simulink model "hmapsf"  (R2020a)
settings: Solver=FixedStepAuto  StartTime=0.0  StopTime=1000000000000000000  FixedStep=tstep  RelTol=1e-3
model workspace (MAT data in the model file):
  IC_x0 = Simulink.Signal
  IC_x0.DataType = 'auto'
  IC_x0.Dimensions = -1
  IC_x0.DimensionsMode = 'auto'
  IC_x0.Complexity = 'auto'
  IC_x0.SampleTime = -1
  IC_x0.SamplingMode = 'auto'
  IC_x1 = Simulink.Signal
  IC_x1.DataType = 'auto'
  IC_x1.Dimensions = -1
  IC_x1.DimensionsMode = 'auto'
  IC_x1.Complexity = 'auto'
  IC_x1.SampleTime = -1
  IC_x1.SamplingMode = 'auto'
  IC_y1 = Simulink.Signal
  IC_y1.DataType = 'auto'
  IC_y1.Dimensions = -1
  IC_y1.DimensionsMode = 'auto'
  IC_y1.Complexity = 'auto'
  IC_y1.SampleTime = -1
  IC_y1.SamplingMode = 'auto'
  contsim_time = Simulink.Signal
  contsim_time.DataType = 'double'
  contsim_time.Dimensions = [1 1]
  contsim_time.DimensionsMode = 'auto'
  contsim_time.Complexity = 'real'
  contsim_time.SampleTime = -1
  contsim_time.SamplingMode = 'auto'
  ip = Simulink.Signal
  ip.DataType = 'double'
  ip.Dimensions = [1 2]
  ip.DimensionsMode = 'auto'
  ip.Complexity = 'auto'
  ip.SampleTime = -1
  ip.SamplingMode = 'auto'
  ip.InitialValue = '[0 0]'
  newnode = Simulink.Signal
  newnode.DataType = 'double'
  newnode.Dimensions = [1 2]
  newnode.DimensionsMode = 'auto'
  newnode.Complexity = 'real'
  newnode.SampleTime = -1
  newnode.SamplingMode = 'auto'
  newnode.InitialValue = '[0 0]'
  szxx1 = Simulink.Signal
  szxx1.DataType = 'double'
  szxx1.Dimensions = [1 1]
  szxx1.DimensionsMode = 'auto'
  szxx1.Complexity = 'real'
  szxx1.SampleTime = -1
  szxx1.SamplingMode = 'auto'
  szxx1.InitialValue = '0'
values from neighbouring files (symbols this model uses):
  H = struct    [hmapsf_Initializ.m]
  IC_theta0 = gamma_1+IC_theta1    (= 4.71238898038)    [hmapsf_Initializ.m]
  IC_theta1 = (3*pi)/2    (= 4.71238898038)    [hmapsf_Initializ.m]
  IC_x0 = IC_x0f-L_0f*cos(IC_theta0)    [hmapsf_Initializ.m]
  IC_x1 = 0    [hmapsf_Initializ.m]
  IC_y0 = IC_y0f-L_0f*sin(IC_theta0)    [hmapsf_Initializ.m]
  IC_y1 = 0    [hmapsf_Initializ.m]
  indsimtime = 300    [hmapsf_Initializ.m]
  L_0b = 0.48    [hmapsf_Initializ.m]
  L_0f = 3.8    [hmapsf_Initializ.m]
  L_1f = 7.21    [hmapsf_Initializ.m]
  LD = 10    [hmapsf_Initializ.m]
  tn = zeros(1,12)    [hmapsf_Initializ.m]
  tstep = 0.2    [hmapsf_Initializ.m]
undefined symbols (not defined in the file or in its folder): DiscIntNeverNeededParam
libraries: simulink x1
settings Model: PauseTimes=0  OrderedModelArguments=off  Creator=giridhar  LastModifiedBy=giridhar
settings SolverCC: AlgebraicLoopSolver=LineSearch
settings DebuggingCC: SFUnusedDataAndEventsDiag=none  UnderSpecifiedDimensionMsg=warning

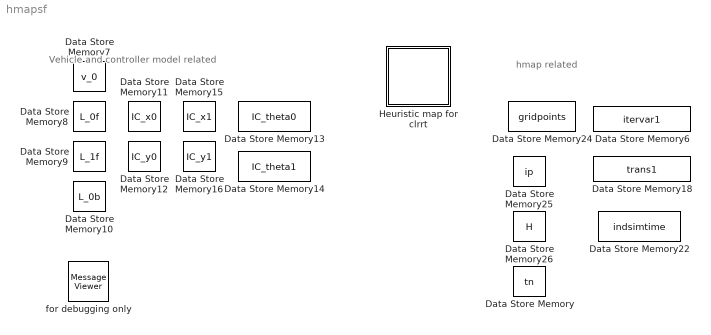
== system hmapsf ==
  note: Vehicle and controller model related
  note: hmap related
  Data Store Memory : DataStoreMemory  DataStoreName=tn  ReadBeforeWriteMsg=warning  WriteAfterWriteMsg=warning  WriteAfterReadMsg=warning  InitialValue=tn  VectorParams1D=off  ShowAdditionalParam=off  OutDataTypeStr=double
  Data Store Memory10 : DataStoreMemory  DataStoreName=L_0b  ReadBeforeWriteMsg=warning  WriteAfterWriteMsg=warning  WriteAfterReadMsg=warning  InitialValue=0.48  VectorParams1D=off  ShowAdditionalParam=off  OutDataTypeStr=double  Dimensions=[1 1]
  Data Store Memory11 : DataStoreMemory  DataStoreName=IC_x0  ReadBeforeWriteMsg=warning  WriteAfterWriteMsg=warning  WriteAfterReadMsg=warning  VectorParams1D=off  ShowAdditionalParam=off  OutDataTypeStr=double  Dimensions=[1 1]  StateMustResolveToSignalObject=on
  Data Store Memory12 : DataStoreMemory  DataStoreName=IC_y0  ReadBeforeWriteMsg=warning  WriteAfterWriteMsg=warning  WriteAfterReadMsg=warning  VectorParams1D=off  ShowAdditionalParam=off  OutDataTypeStr=double  Dimensions=[1 1]
  Data Store Memory13 : DataStoreMemory  DataStoreName=IC_theta0  ReadBeforeWriteMsg=warning  WriteAfterWriteMsg=warning  WriteAfterReadMsg=warning  VectorParams1D=off  ShowAdditionalParam=off  OutDataTypeStr=double  Dimensions=[1 1]
  Data Store Memory14 : DataStoreMemory  DataStoreName=IC_theta1  ReadBeforeWriteMsg=warning  WriteAfterWriteMsg=warning  WriteAfterReadMsg=warning  VectorParams1D=off  ShowAdditionalParam=off  OutDataTypeStr=double  Dimensions=[1 1]
  Data Store Memory15 : DataStoreMemory  DataStoreName=IC_x1  ReadBeforeWriteMsg=warning  WriteAfterWriteMsg=warning  WriteAfterReadMsg=warning  VectorParams1D=off  ShowAdditionalParam=off  OutDataTypeStr=double  Dimensions=[1 1]  StateMustResolveToSignalObject=on
  Data Store Memory16 : DataStoreMemory  DataStoreName=IC_y1  ReadBeforeWriteMsg=warning  WriteAfterWriteMsg=warning  WriteAfterReadMsg=warning  VectorParams1D=off  ShowAdditionalParam=off  OutDataTypeStr=double  Dimensions=[1 1]  StateMustResolveToSignalObject=on
  Data Store Memory18 : DataStoreMemory  DataStoreName=trans1  ReadBeforeWriteMsg=warning  WriteAfterWriteMsg=warning  WriteAfterReadMsg=warning  VectorParams1D=off  ShowAdditionalParam=off  OutDataTypeStr=double
  Data Store Memory22 : DataStoreMemory  DataStoreName=indsimtime  ReadBeforeWriteMsg=warning  WriteAfterWriteMsg=warning  WriteAfterReadMsg=warning  InitialValue=indsimtime  ShowAdditionalParam=off  OutDataTypeStr=double
  Data Store Memory24 : DataStoreMemory  DataStoreName=gridpoints  ReadBeforeWriteMsg=warning  WriteAfterWriteMsg=warning  WriteAfterReadMsg=warning  InitialValue=gridpoints  VectorParams1D=off  ShowAdditionalParam=off  OutDataTypeStr=double
  Data Store Memory25 : DataStoreMemory  DataStoreName=ip  ReadBeforeWriteMsg=warning  WriteAfterWriteMsg=warning  WriteAfterReadMsg=warning  InitialValue=[0 0]  VectorParams1D=off  ShowAdditionalParam=off  OutDataTypeStr=double  Dimensions=[1 2]  StateMustResolveToSignalObject=on
  Data Store Memory26 : DataStoreMemory  DataStoreName=H  ReadBeforeWriteMsg=warning  WriteAfterWriteMsg=warning  WriteAfterReadMsg=warning  InitialValue=H  VectorParams1D=off  ShowAdditionalParam=off  OutDataTypeStr=Bus: slBus1
  Data Store Memory6 : DataStoreMemory  DataStoreName=itervar1  ReadBeforeWriteMsg=warning  WriteAfterWriteMsg=warning  WriteAfterReadMsg=warning  VectorParams1D=off  ShowAdditionalParam=off  OutDataTypeStr=double
  Data Store Memory7 : DataStoreMemory  DataStoreName=v_0  ReadBeforeWriteMsg=warning  WriteAfterWriteMsg=warning  WriteAfterReadMsg=warning  InitialValue=v_0  VectorParams1D=off  ShowAdditionalParam=off  OutDataTypeStr=double  Dimensions=[1 1]
  Data Store Memory8 : DataStoreMemory  DataStoreName=L_0f  ReadBeforeWriteMsg=warning  WriteAfterWriteMsg=warning  WriteAfterReadMsg=warning  InitialValue=3.8  VectorParams1D=off  ShowAdditionalParam=off  OutDataTypeStr=double  Dimensions=[1 1]
  Data Store Memory9 : DataStoreMemory  DataStoreName=L_1f  ReadBeforeWriteMsg=warning  WriteAfterWriteMsg=warning  WriteAfterReadMsg=warning  InitialValue=7.21  VectorParams1D=off  ShowAdditionalParam=off  OutDataTypeStr=double  Dimensions=[1 1]
  Heuristic map for clrrt : Stateflow chart  TreatAsAtomicUnit=on
  for debugging only : MessageViewer  History=1000  SavedRootId=#

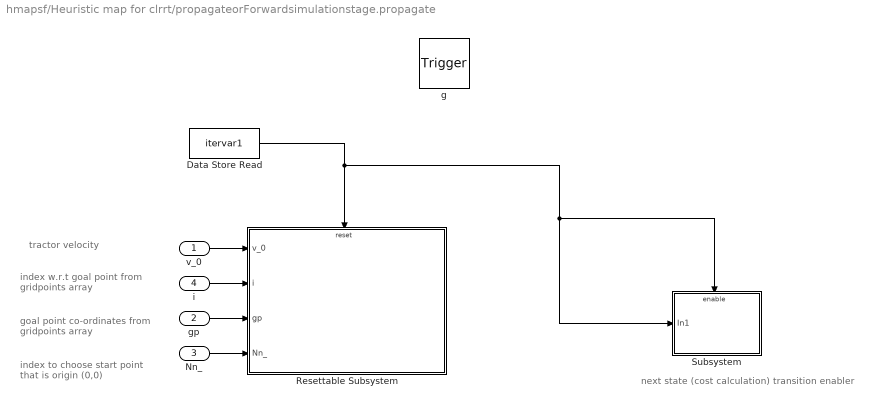
== system hmapsf/Heuristic map for clrrt/propagateorForwardsimulationstage.propagate ==
  note: index w.r.t goal point from
      | gridpoints array
  note: index to choose start point
      | that is origin (0,0)
  note: goal point co-ordinates from
      | gridpoints array
  note: tractor velocity
  note: next state (cost calculation) transition enabler
  v_0 : Inport  OutDataTypeStr=double  PortDimensions=1
  gp : Inport  Port=2  OutMin=1  OutMax=2  OutDataTypeStr=double  PortDimensions=[1 3]
  Nn_ : Inport  Port=3  OutDataTypeStr=double  PortDimensions=1
  i : Inport  Port=4  OutDataTypeStr=double  PortDimensions=1
  g : TriggerPort  TriggerType=function-call  VariantControl=(inherit)  SampleTime=0.2
      settings: CopyFcn=Stateflow.SLINSF.SimulinkMan.removeBlockPreDeleteFcn  PreDeleteFcn=Stateflow.SLINSF.SimulinkMan.unsafePredeleteFcn
  Data Store Read : DataStoreRead  DataStoreName=itervar1
  Resettable Subsystem : Subsystem  Priority=1  TreatAsAtomicUnit=on
  Subsystem : Subsystem  Priority=2
  wires:
  gp/1 -> Resettable Subsystem/3(gp)
  v_0/1 -> Resettable Subsystem/1(v_0)
  Nn_/1 -> Resettable Subsystem/4(Nn_)
  i/1 -> Resettable Subsystem/2(i)
  Data Store Read/1 -> Subsystem/Enable, Subsystem/1(In1), Resettable Subsystem/Reset

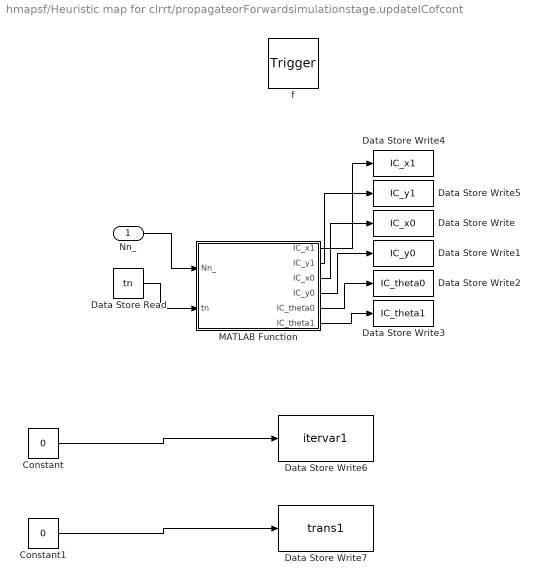
== system hmapsf/Heuristic map for clrrt/propagateorForwardsimulationstage.updateICofcont ==
  Nn_ : Inport  OutDataTypeStr=double  PortDimensions=1
  f : TriggerPort  TriggerType=function-call  VariantControl=(inherit)
      settings: CopyFcn=Stateflow.SLINSF.SimulinkMan.removeBlockPreDeleteFcn  PreDeleteFcn=Stateflow.SLINSF.SimulinkMan.unsafePredeleteFcn
  Constant : Constant  Value=0
  Constant1 : Constant  Value=0
  Data Store Read : DataStoreRead  DataStoreName=tn
  Data Store Write : DataStoreWrite  DataStoreName=IC_x0
  Data Store Write1 : DataStoreWrite  DataStoreName=IC_y0
  Data Store Write2 : DataStoreWrite  DataStoreName=IC_theta0
  Data Store Write3 : DataStoreWrite  DataStoreName=IC_theta1
  Data Store Write4 : DataStoreWrite  DataStoreName=IC_x1
  Data Store Write5 : DataStoreWrite  DataStoreName=IC_y1
  Data Store Write6 : DataStoreWrite  DataStoreName=itervar1
  Data Store Write7 : DataStoreWrite  DataStoreName=trans1
  MATLAB Function : MATLAB Function  TreatAsAtomicUnit=on
  wires:
  Nn_/1 -> MATLAB Function/1(Nn_)
  Data Store Read/1 -> MATLAB Function/2(tn)
  MATLAB Function/6(IC_theta1) -> Data Store Write3/1
  MATLAB Function/5(IC_theta0) -> Data Store Write2/1
  MATLAB Function/4(IC_y0) -> Data Store Write1/1
  MATLAB Function/3(IC_x0) -> Data Store Write/1
  MATLAB Function/2(IC_y1) -> Data Store Write5/1
  MATLAB Function/1(IC_x1) -> Data Store Write4/1
  Constant/1 -> Data Store Write6/1
  Constant1/1 -> Data Store Write7/1

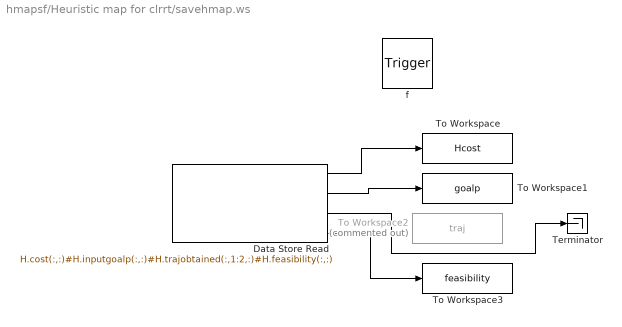
== system hmapsf/Heuristic map for clrrt/savehmap.ws ==
  f : TriggerPort  TriggerType=function-call  VariantControl=(inherit)
      settings: CopyFcn=Stateflow.SLINSF.SimulinkMan.removeBlockPreDeleteFcn  PreDeleteFcn=Stateflow.SLINSF.SimulinkMan.unsafePredeleteFcn
  Data Store Read : DataStoreRead  DataStoreName=H  DataStoreElements=H.cost(:,:)#H.inputgoalp(:,:)#H.trajobtained(:,1:2,:)#H.feasibility(:,:)
  Terminator : Terminator
  To Workspace : ToWorkspace  VariableName=Hcost  SaveFormat=Structure  SampleTime=-1
  To Workspace1 : ToWorkspace  VariableName=goalp  SaveFormat=Timeseries  SampleTime=-1
  To Workspace2 : ToWorkspace  Commented=on  VariableName=traj  SaveFormat=Structure  SampleTime=-1
  To Workspace3 : ToWorkspace  VariableName=feasibility  SaveFormat=Structure  SampleTime=-1
  wires:
  Data Store Read/1 -> To Workspace/1
  Data Store Read/2 -> To Workspace1/1
  Data Store Read/3 -> Terminator/1
  Data Store Read/4 -> To Workspace3/1

== system hmapsf/Heuristic map for clrrt/stop ==
  f : TriggerPort  TriggerType=function-call  VariantControl=(inherit)
      settings: CopyFcn=Stateflow.SLINSF.SimulinkMan.removeBlockPreDeleteFcn  PreDeleteFcn=Stateflow.SLINSF.SimulinkMan.unsafePredeleteFcn
  Constant : Constant
  Stop Simulation : Stop
  wires:
  Constant/1 -> Stop Simulation/1

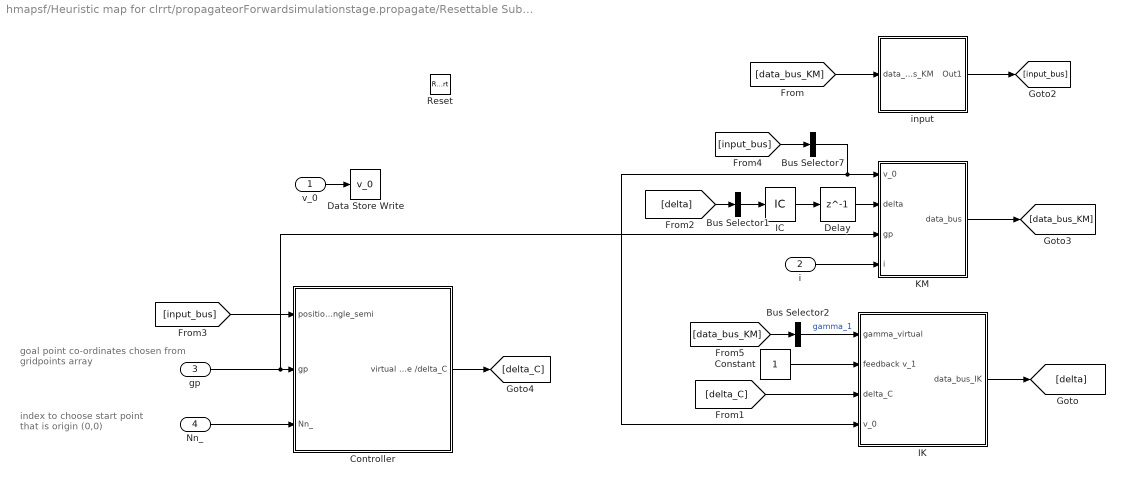
== system hmapsf/Heuristic map for clrrt/propagateorForwardsimulationstage.propagate/Resettable Subsystem ==
  note: goal point co-ordinates chosen from
      | gridpoints array
  note: index to choose start point
      | that is origin (0,0)
  v_0 : Inport  OutDataTypeStr=double  PortDimensions=1
  i : Inport  Port=2  OutDataTypeStr=double  PortDimensions=1
  gp : Inport  Port=3  OutMin=1  OutMax=2  OutDataTypeStr=double  PortDimensions=[1 3]
  Nn_ : Inport  Port=4  OutDataTypeStr=double  PortDimensions=1
  Reset : ResetPort  DisableCoverage=on  ResetTriggerType=level  PropagateVarSize=During execution
  Bus Selector1 : BusSelector  OutputSignals=angle.steering_angle  OutputAsBus=on
  Bus Selector2 : BusSelector  OutputSignals=angle.articulation_angle  OutputAsBus=on
  Bus Selector7 : BusSelector  OutputSignals=u_0  OutputAsBus=on
  Constant : Constant
  Controller : Subsystem
  Data Store Write : DataStoreWrite  DataStoreName=v_0
  Delay : Delay  DelayLength=1
  IC : InitialCondition  Value=0
  IK : Subsystem  SystemSampleTime=0.8
  KM : Subsystem  SystemSampleTime=0.8
  input : Subsystem
  wires:
  [data_bus_KM] -> Bus Selector2/1
  input/1(Out1) -> [input_bus]
  [delta_C] -> IK/3(delta_C)
  Bus Selector7/1 -> IK/4(v_0), KM/1(v_0)
  [delta] -> Bus Selector1/1
  Nn_/1 -> Controller/3(Nn_)
  i/1 -> KM/4(i)
  Delay/1 -> KM/2(delta)
  Constant/1 -> IK/2(feedback v_1)
  IC/1 -> Delay/1
  KM/1(data_bus) -> [data_bus_KM]
  Bus Selector2/1 -> IK/1(gamma_virtual)  "gamma_1"
  Bus Selector1/1 -> IC/1
  v_0/1 -> Data Store Write/1
  IK/1(data_bus_IK) -> [delta]
  [input_bus] -> Bus Selector7/1
  [data_bus_KM] -> input/1(data_bus_KM)
  [input_bus] -> Controller/1(positions_yawangle_semi)
  gp/1 -> Controller/2(gp), KM/3(gp)
  Controller/1(virtual steer angle /delta_C) -> [delta_C]

== system hmapsf/Heuristic map for clrrt/propagateorForwardsimulationstage.propagate/Subsystem ==
  In1 : Inport
  Enable : EnablePort  StatesWhenEnabling=reset
  Subsystem : Subsystem  Priority=2
  wires:
  In1/1 -> Subsystem/1(In1)

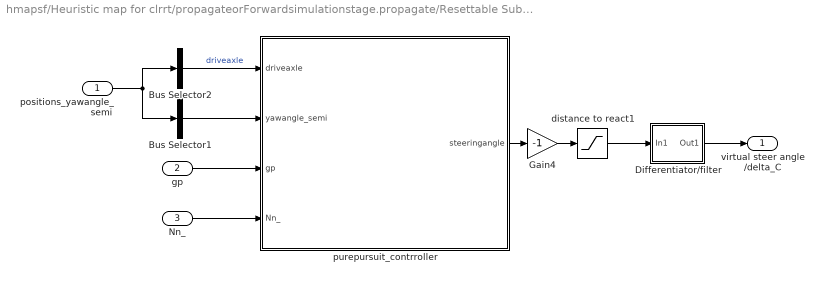
== system hmapsf/Heuristic map for clrrt/propagateorForwardsimulationstage.propagate/Resettable Subsystem/Controller ==
  positions_yawangle_semi : Inport
  gp : Inport  Port=2
  Nn_ : Inport  Port=3
  Bus Selector1 : BusSelector  OutputSignals=yawangle_semi  OutputAsBus=on
  Bus Selector2 : BusSelector  OutputSignals=positions  OutputAsBus=on
  Differentiator/filter : Subsystem  mask{ts=13.5}
      mask prompts: ts "response_time"
      mask init:
      | c=(3*pi/ts)^2;
  Gain4 : Gain  Gain=-1
  distance to react1 : Saturate  UpperLimit=1  LowerLimit=-1
  purepursuit_contrroller : Subsystem
  virtual steer angle /delta_C : Outport  PortDimensions=[1,1]  VectorParamsAs1DForOutWhenUnconnected=off
  wires:
  distance to react1/1 -> Differentiator/filter/1(In1)
  purepursuit_contrroller/1(steeringangle) -> Gain4/1
  Bus Selector2/1 -> purepursuit_contrroller/1(driveaxle)  "driveaxle"
  positions_yawangle_semi/1 -> Bus Selector1/1, Bus Selector2/1
  gp/1 -> purepursuit_contrroller/3(gp)
  Nn_/1 -> purepursuit_contrroller/4(Nn_)
  Gain4/1 -> distance to react1/1
  Bus Selector1/1 -> purepursuit_contrroller/2(yawangle_semi)
  Differentiator/filter/1(Out1) -> virtual steer angle /delta_C/1

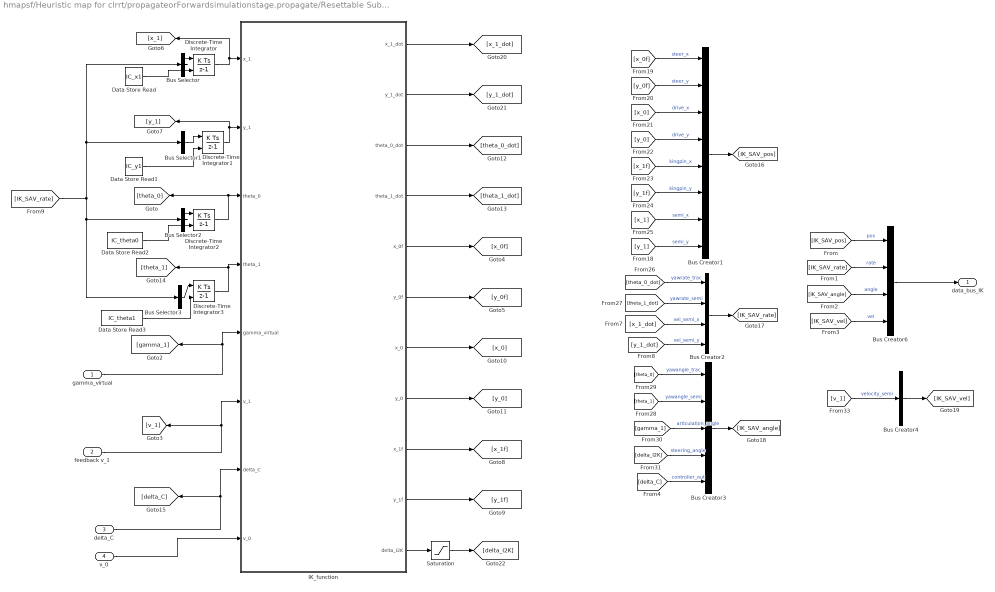
== system hmapsf/Heuristic map for clrrt/propagateorForwardsimulationstage.propagate/Resettable Subsystem/IK ==
  gamma_virtual : Inport
  feedback v_1 : Inport  Port=2
  delta_C : Inport  Port=3
  v_0 : Inport  Port=4
  Bus Creator1 : BusCreator  Inputs=8
  Bus Creator2 : BusCreator  Inputs=4
  Bus Creator3 : BusCreator  Inputs=5
  Bus Creator4 : BusCreator  Inputs=1
  Bus Creator6 : BusCreator  Inputs=4
  Bus Selector : BusSelector  OutputSignals=vel_semi_x  OutputAsBus=on
  Bus Selector1 : BusSelector  OutputSignals=vel_semi_y  OutputAsBus=on
  Bus Selector2 : BusSelector  OutputSignals=yawrate_trac  OutputAsBus=on
  Bus Selector3 : BusSelector  OutputSignals=yawrate_semi  OutputAsBus=on
  Data Store Read : DataStoreRead  DataStoreName=IC_x1
  Data Store Read1 : DataStoreRead  DataStoreName=IC_y1
  Data Store Read2 : DataStoreRead  DataStoreName=IC_theta0
  Data Store Read3 : DataStoreRead  DataStoreName=IC_theta1
  Discrete-Time Integrator : DiscreteIntegrator  InitialConditionSource=external  InitialCondition=IC_x1  SampleTime=-1  ICPrevOutput=DiscIntNeverNeededParam  ICPrevScaledInput=DiscIntNeverNeededParam
  Discrete-Time Integrator1 : DiscreteIntegrator  InitialConditionSource=external  InitialCondition=IC_y1  SampleTime=-1  ICPrevOutput=DiscIntNeverNeededParam  ICPrevScaledInput=DiscIntNeverNeededParam
  Discrete-Time Integrator2 : DiscreteIntegrator  InitialConditionSource=external  InitialCondition=IC_theta0  SampleTime=-1  ICPrevOutput=DiscIntNeverNeededParam  ICPrevScaledInput=DiscIntNeverNeededParam
  Discrete-Time Integrator3 : DiscreteIntegrator  InitialConditionSource=external  InitialCondition=IC_theta1  SampleTime=-1  ICPrevOutput=DiscIntNeverNeededParam  ICPrevScaledInput=DiscIntNeverNeededParam
  IK_function : MATLAB Function  TreatAsAtomicUnit=on
  Saturation : Saturate  UpperLimit=0.7  LowerLimit=-0.7
  data_bus_IK : Outport  VectorParamsAs1DForOutWhenUnconnected=off
  wires:
  IK_function/7(x_0) -> [x_0]
  IK_function/8(y_0) -> [y_0]
  IK_function/1(x_1_dot) -> [x_1_dot]
  IK_function/3(theta_0_dot) -> [theta_0_dot]
  IK_function/4(theta_1_dot) -> [theta_1_dot]
  IK_function/10(y_1f) -> [y_1f]
  IK_function/9(x_1f) -> [x_1f]
  Discrete-Time Integrator/1 -> [x_1], IK_function/1(x_1)
  Discrete-Time Integrator1/1 -> [y_1], IK_function/2(y_1)
  gamma_virtual/1 -> [gamma_1], IK_function/5(gamma_virtual)
  IK_function/2(y_1_dot) -> [y_1_dot]
  Discrete-Time Integrator3/1 -> IK_function/4(theta_1), [theta_1]
  IK_function/5(x_0f) -> [x_0f]
  IK_function/6(y_0f) -> [y_0f]
  [y_0f] -> Bus Creator1/2  "steer_y"
  [x_1f] -> Bus Creator1/5  "kingpin_x"
  Bus Creator6/1 -> data_bus_IK/1
  [v_1] -> Bus Creator4/1  "velocity_semi"
  [x_0] -> Bus Creator1/3  "drive_x"
  [y_1f] -> Bus Creator1/6  "kingpin_y"
  [x_0f] -> Bus Creator1/1  "steer_x"
  [y_0] -> Bus Creator1/4  "drive_y"
  Bus Creator3/1 -> [IK_SAV_angle]
  [theta_0_dot] -> Bus Creator2/1  "yawrate_trac"
  [theta_1_dot] -> Bus Creator2/2  "yawrate_semi"
  Discrete-Time Integrator2/1 -> [theta_0], IK_function/3(theta_0)
  [IK_SAV_rate] -> Bus Selector/1, Bus Selector1/1, Bus Selector3/1, Bus Selector2/1
  Bus Creator2/1 -> [IK_SAV_rate]
  Bus Creator1/1 -> [IK_SAV_pos]
  [delta_I2K] -> Bus Creator3/4  "steering_angle"
  [gamma_1] -> Bus Creator3/3  "articulation_angle"
  Bus Creator4/1 -> [IK_SAV_vel]
  [theta_1] -> Bus Creator3/2  "yawangle_semi"
  [IK_SAV_rate] -> Bus Creator6/2  "rate"
  [theta_0] -> Bus Creator3/1  "yawangle_trac"
  [IK_SAV_pos] -> Bus Creator6/1  "pos"
  [IK_SAV_angle] -> Bus Creator6/3  "angle"
  [IK_SAV_vel] -> Bus Creator6/4  "vel"
  Bus Selector3/1 -> Discrete-Time Integrator3/1
  Bus Selector2/1 -> Discrete-Time Integrator2/1
  Bus Selector/1 -> Discrete-Time Integrator/1
  Bus Selector1/1 -> Discrete-Time Integrator1/1
  [y_1_dot] -> Bus Creator2/4  "vel_semi_y"
  [x_1_dot] -> Bus Creator2/3  "vel_semi_x"
  IK_function/11(delta_I2K) -> Saturation/1
  [delta_C] -> Bus Creator3/5  "controller_out"
  feedback v_1/1 -> [v_1], IK_function/6(v_1)
  Saturation/1 -> [delta_I2K]
  [y_1] -> Bus Creator1/8  "semi_y"
  [x_1] -> Bus Creator1/7  "semi_x"
  Data Store Read3/1 -> Discrete-Time Integrator3/2
  Data Store Read2/1 -> Discrete-Time Integrator2/2
  Data Store Read1/1 -> Discrete-Time Integrator1/2
  Data Store Read/1 -> Discrete-Time Integrator/2
  v_0/1 -> IK_function/8(v_0)
  delta_C/1 -> IK_function/7(delta_C), [delta_C]

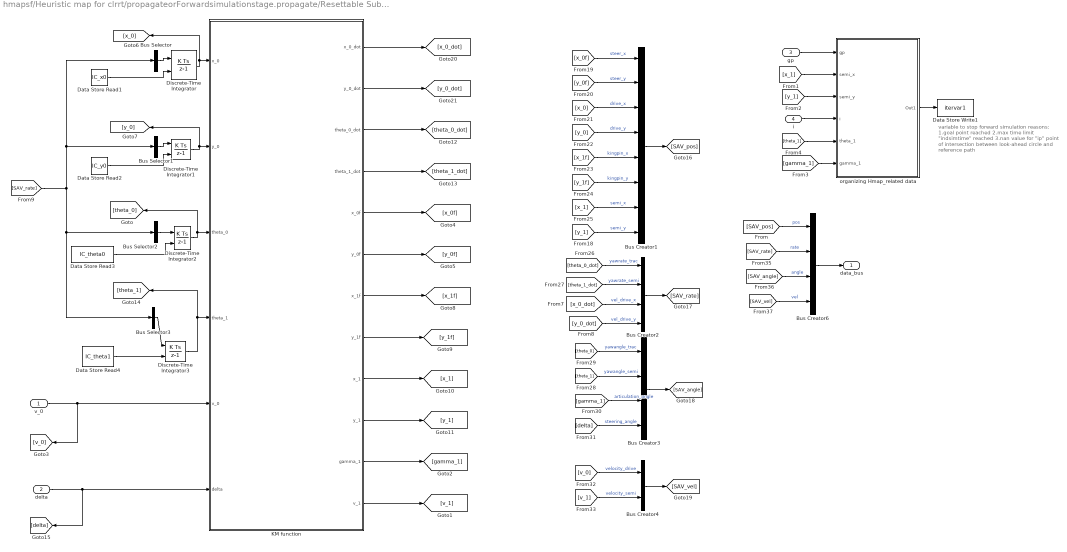
== system hmapsf/Heuristic map for clrrt/propagateorForwardsimulationstage.propagate/Resettable Subsystem/KM ==
  note: variable to stop forward simulation
      | reasons:
      | 1.goal point reached
      | 2.max time limit "indsimtime" reached
      | 3.nan value for "ip" point of intersection
      | between look-ahead circle and reference path
  v_0 : Inport
  delta : Inport  Port=2
  gp : Inport  Port=3
  i : Inport  Port=4  OutDataTypeStr=double
  Bus Creator1 : BusCreator  Inputs=8
  Bus Creator2 : BusCreator  Inputs=4
  Bus Creator3 : BusCreator  Inputs=4
  Bus Creator4 : BusCreator  Inputs=2
  Bus Creator6 : BusCreator  Inputs=4
  Bus Selector : BusSelector  OutputSignals=vel_drive_x  OutputAsBus=on
  Bus Selector1 : BusSelector  OutputSignals=vel_drive_y  OutputAsBus=on
  Bus Selector2 : BusSelector  OutputSignals=yawrate_trac  OutputAsBus=on
  Bus Selector3 : BusSelector  OutputSignals=yawrate_semi  OutputAsBus=on
  Data Store Read1 : DataStoreRead  DataStoreName=IC_x0
  Data Store Read2 : DataStoreRead  DataStoreName=IC_y0
  Data Store Read3 : DataStoreRead  DataStoreName=IC_theta0
  Data Store Read4 : DataStoreRead  DataStoreName=IC_theta1
  Data Store Write1 : DataStoreWrite  DataStoreName=itervar1
  Discrete-Time Integrator : DiscreteIntegrator  InitialConditionSource=external  InitialCondition=IC_x0  SampleTime=-1  ICPrevOutput=DiscIntNeverNeededParam  ICPrevScaledInput=DiscIntNeverNeededParam
  Discrete-Time Integrator1 : DiscreteIntegrator  InitialConditionSource=external  InitialCondition=IC_y0  SampleTime=-1  ICPrevOutput=DiscIntNeverNeededParam  ICPrevScaledInput=DiscIntNeverNeededParam
  Discrete-Time Integrator2 : DiscreteIntegrator  InitialConditionSource=external  InitialCondition=IC_theta0  SampleTime=-1  ICPrevOutput=DiscIntNeverNeededParam  ICPrevScaledInput=DiscIntNeverNeededParam
  Discrete-Time Integrator3 : DiscreteIntegrator  InitialConditionSource=external  InitialCondition=IC_theta1  SampleTime=-1  ICPrevOutput=DiscIntNeverNeededParam  ICPrevScaledInput=DiscIntNeverNeededParam
  KM function : MATLAB Function  TreatAsAtomicUnit=on
  "organizing Hmap_related data " : Subsystem
  data_bus : Outport  VectorParamsAs1DForOutWhenUnconnected=off
  wires:
  KM function/9(x_1) -> [x_1]
  KM function/10(y_1) -> [y_1]
  KM function/1(x_0_dot) -> [x_0_dot]
  KM function/3(theta_0_dot) -> [theta_0_dot]
  KM function/4(theta_1_dot) -> [theta_1_dot]
  KM function/8(y_1f) -> [y_1f]
  KM function/7(x_1f) -> [x_1f]
  Discrete-Time Integrator/1 -> KM function/1(x_0), [x_0]
  Discrete-Time Integrator1/1 -> KM function/2(y_0), [y_0]
  KM function/11(gamma_1) -> [gamma_1]
  KM function/2(y_0_dot) -> [y_0_dot]
  delta/1 -> [delta], KM function/6(delta)
  Discrete-Time Integrator3/1 -> [theta_1], KM function/4(theta_1)
  KM function/5(x_0f) -> [x_0f]
  KM function/6(y_0f) -> [y_0f]
  v_0/1 -> [v_0], KM function/5(v_0)
  [y_0f] -> Bus Creator1/2  "steer_y"
  [x_1f] -> Bus Creator1/5  "kingpin_x"
  Bus Creator6/1 -> data_bus/1
  [v_1] -> Bus Creator4/2  "velocity_semi"
  [x_0] -> Bus Creator1/3  "drive_x"
  [y_1f] -> Bus Creator1/6  "kingpin_y"
  [x_0f] -> Bus Creator1/1  "steer_x"
  [y_0] -> Bus Creator1/4  "drive_y"
  Bus Creator3/1 -> [SAV_angle]
  [v_0] -> Bus Creator4/1  "velocity_drive"
  [theta_0_dot] -> Bus Creator2/1  "yawrate_trac"
  [theta_1_dot] -> Bus Creator2/2  "yawrate_semi"
  Discrete-Time Integrator2/1 -> [theta_0], KM function/3(theta_0)
  [SAV_rate] -> Bus Selector/1, Bus Selector1/1, Bus Selector3/1, Bus Selector2/1
  Bus Creator2/1 -> [SAV_rate]
  Bus Creator1/1 -> [SAV_pos]
  [delta] -> Bus Creator3/4  "steering_angle"
  [gamma_1] -> Bus Creator3/3  "articulation_angle"
  Bus Creator4/1 -> [SAV_vel]
  [theta_1] -> Bus Creator3/2  "yawangle_semi"
  [SAV_rate] -> Bus Creator6/2  "rate"
  [theta_0] -> Bus Creator3/1  "yawangle_trac"
  [SAV_pos] -> Bus Creator6/1  "pos"
  [SAV_angle] -> Bus Creator6/3  "angle"
  [SAV_vel] -> Bus Creator6/4  "vel"
  Bus Selector3/1 -> Discrete-Time Integrator3/1
  Bus Selector2/1 -> Discrete-Time Integrator2/1
  Bus Selector/1 -> Discrete-Time Integrator/1
  Bus Selector1/1 -> Discrete-Time Integrator1/1
  [y_0_dot] -> Bus Creator2/4  "vel_drive_y"
  [x_0_dot] -> Bus Creator2/3  "vel_drive_x"
  KM function/12(v_1) -> [v_1]
  [x_1] -> Bus Creator1/7  "semi_x"
  [y_1] -> Bus Creator1/8  "semi_y"
  Data Store Read4/1 -> Discrete-Time Integrator3/2
  Data Store Read2/1 -> Discrete-Time Integrator1/2
  Data Store Read3/1 -> Discrete-Time Integrator2/2
  gp/1 -> "organizing Hmap_related data "/1(gp)
  i/1 -> "organizing Hmap_related data "/4(i)
  "organizing Hmap_related data "/1(Out1) -> Data Store Write1/1
  [theta_1] -> "organizing Hmap_related data "/5(theta_1)
  [y_1] -> "organizing Hmap_related data "/3(semi_y)
  [x_1] -> "organizing Hmap_related data "/2(semi_x)
  [gamma_1] -> "organizing Hmap_related data "/6(gamma_1)
  Data Store Read1/1 -> Discrete-Time Integrator/2

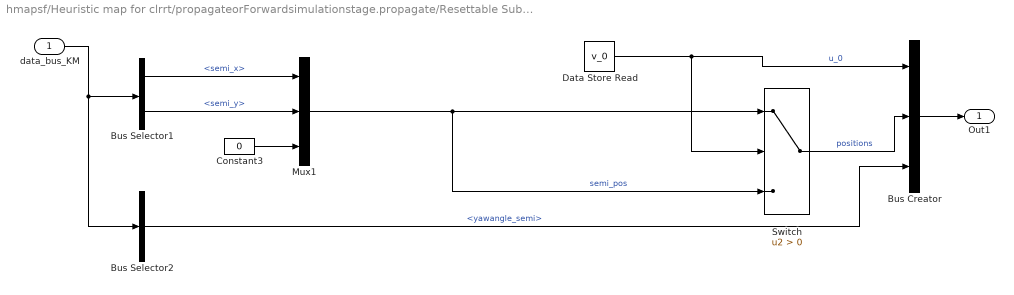
== system hmapsf/Heuristic map for clrrt/propagateorForwardsimulationstage.propagate/Resettable Subsystem/input ==
  data_bus_KM : Inport
  Bus Creator : BusCreator  Inputs=3
  Bus Selector1 : BusSelector  OutputSignals=pos.semi_x,pos.semi_y
  Bus Selector2 : BusSelector  OutputSignals=angle.yawangle_semi
  Constant3 : Constant  Value=0
  Data Store Read : DataStoreRead  DataStoreName=v_0
  Mux1 : Mux  Inputs=3
  Switch : Switch  Criteria=u2 > Threshold
  Out1 : Outport  VectorParamsAs1DForOutWhenUnconnected=off
  wires:
  Data Store Read/1 -> Switch/2, Bus Creator/1  "u_0"
  Bus Creator/1 -> Out1/1
  Constant3/1 -> Mux1/3
  data_bus_KM/1 -> Bus Selector2/1, Bus Selector1/1
  Bus Selector1/1 -> Mux1/1  "<semi_x>"
  Bus Selector1/2 -> Mux1/2  "<semi_y>"
  Mux1/1 -> Switch/1, Switch/3  "semi_pos"
  Switch/1 -> Bus Creator/2  "positions"
  Bus Selector2/1 -> Bus Creator/3  "<yawangle_semi>"

== system hmapsf/Heuristic map for clrrt/propagateorForwardsimulationstage.propagate/Subsystem/Subsystem ==
  note: variable for the stateflow transition condition
      | lets the control flow from forward simulation to cost calculation
      | in stateflow chart
  In1 : Inport
  Data Store Write : DataStoreWrite  DataStoreName=trans1
  wires:
  In1/1 -> Data Store Write/1

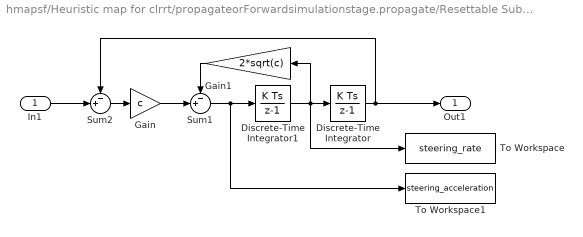
== system hmapsf/Heuristic map for clrrt/propagateorForwardsimulationstage.propagate/Resettable Subsystem/Controller/Differentiator//filter ==
  In1 : Inport
  Discrete-Time Integrator : DiscreteIntegrator  SampleTime=-1  ICPrevOutput=DiscIntNeverNeededParam  ICPrevScaledInput=DiscIntNeverNeededParam
  Discrete-Time Integrator1 : DiscreteIntegrator  SampleTime=-1  ICPrevOutput=DiscIntNeverNeededParam  ICPrevScaledInput=DiscIntNeverNeededParam
  Gain : Gain  Gain=c  SaturateOnIntegerOverflow=on  OutDataTypeStr=Inherit: Same as input  ParamDataTypeStr=Inherit: Same as input
  Gain1 : Gain  Gain=2*sqrt(c)  SaturateOnIntegerOverflow=on  OutDataTypeStr=Inherit: Same as input  ParamDataTypeStr=Inherit: Same as input
  Sum1 : Sum  Inputs=-+|  SaturateOnIntegerOverflow=on
  Sum2 : Sum  Inputs=-+|  SaturateOnIntegerOverflow=on
  To Workspace : ToWorkspace  VariableName=steering_rate  SampleTime=-1
  To Workspace1 : ToWorkspace  VariableName=steering_acceleration  SampleTime=-1
  Out1 : Outport
  wires:
  Discrete-Time Integrator1/1 -> Discrete-Time Integrator/1, To Workspace/1, Gain1/1
  Discrete-Time Integrator/1 -> Out1/1, Sum2/1
  Sum1/1 -> Discrete-Time Integrator1/1, To Workspace1/1
  Sum2/1 -> Gain/1
  In1/1 -> Sum2/2
  Gain1/1 -> Sum1/1
  Gain/1 -> Sum1/2

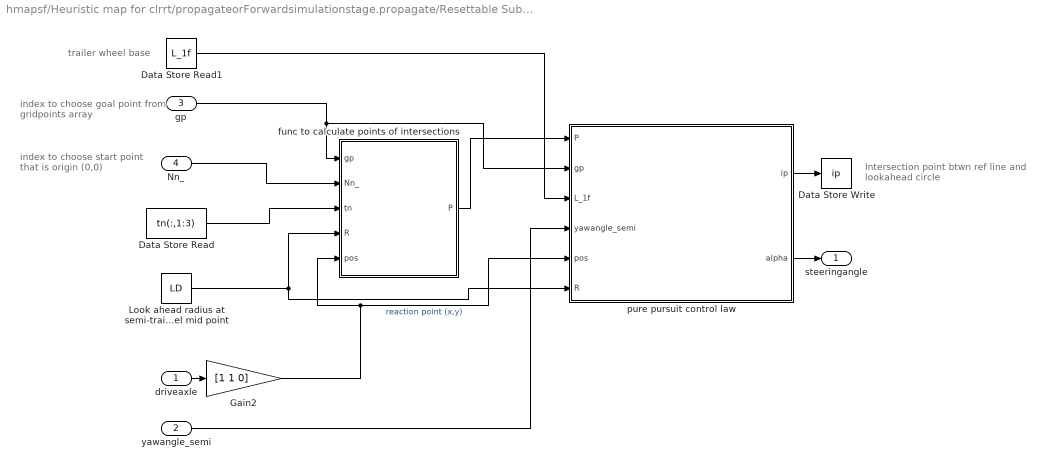
== system hmapsf/Heuristic map for clrrt/propagateorForwardsimulationstage.propagate/Resettable Subsystem/Controller/purepursuit_contrroller ==
  note: index to choose goal point from
      | gridpoints array
  note: trailer wheel base
  note: Intersection point
      | btwn ref line and lookahead circle
  note: index to choose start point
      | that is origin (0,0)
  driveaxle : Inport
  yawangle_semi : Inport  Port=2
  gp : Inport  Port=3
  Nn_ : Inport  Port=4
  Data Store Read : DataStoreRead  DataStoreName=tn  DataStoreElements=tn(:,1:3)
  Data Store Read1 : DataStoreRead  DataStoreName=L_1f
  Data Store Write : DataStoreWrite  DataStoreName=ip
  Gain2 : Gain  Gain=[1 1 0]
  Look ahead radius at semi-trailer axel mid point : Constant  Value=LD
  func to calculate points of intersections : MATLAB Function  TreatAsAtomicUnit=on
  pure pursuit control law : MATLAB Function  TreatAsAtomicUnit=on
  steeringangle : Outport  VectorParamsAs1DForOutWhenUnconnected=off
  wires:
  Data Store Read1/1 -> pure pursuit control law/3(L_1f)
  func to calculate points of intersections/1(P) -> pure pursuit control law/1(P)
  pure pursuit control law/1(ip) -> Data Store Write/1
  Look ahead radius at semi-trailer axel mid point/1 -> func to calculate points of intersections/4(R), pure pursuit control law/6(R)
  pure pursuit control law/2(alpha) -> steeringangle/1
  gp/1 -> func to calculate points of intersections/1(gp), pure pursuit control law/2(gp)
  Gain2/1 -> func to calculate points of intersections/5(pos), pure pursuit control law/5(pos)  "reaction point (x,y)"
  driveaxle/1 -> Gain2/1
  yawangle_semi/1 -> pure pursuit control law/4(yawangle_semi)
  Nn_/1 -> func to calculate points of intersections/2(Nn_)
  Data Store Read/1 -> func to calculate points of intersections/3(tn)

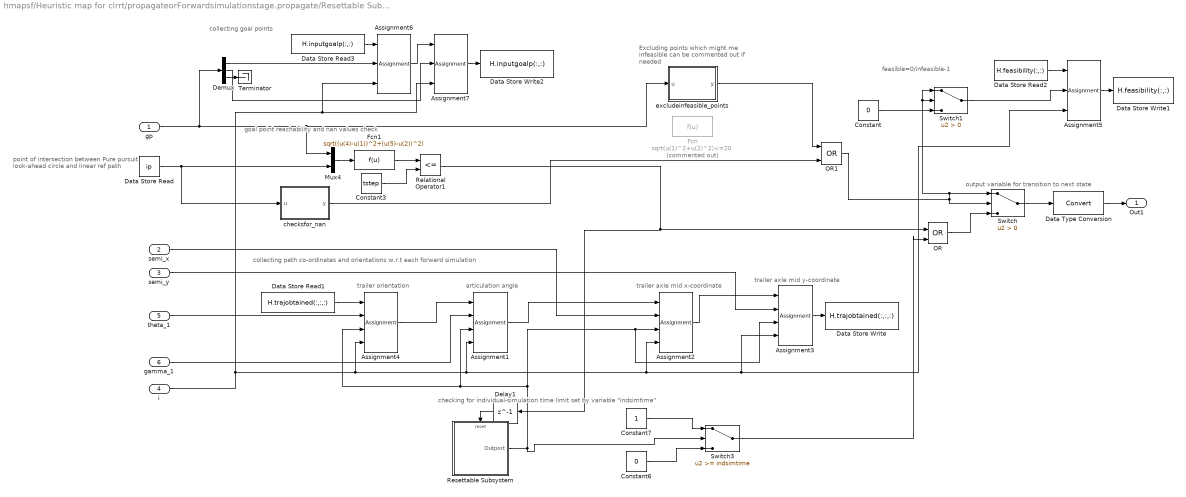
== system hmapsf/Heuristic map for clrrt/propagateorForwardsimulationstage.propagate/Resettable Subsystem/KM/organizing Hmap_related data  ==
  note: checking for individual simulation time limit set by variable "indsimtime"
  note: output variable for transition to next state
  note: Excluding points which might me infeasible can be commented out if needed
  note: collecting path co-ordinates and orientations w.r.t each forward simulation
  note: goal point reachability and nan values check
  note: point of intersection between Pure pursuit
      | look-ahead circle and linear ref path
  note: collecting goal points
  note: feasible=0/infeasible-1
  note: trailer axle mid x-coordinate
  note: trailer orientation
  note: articulation angle
  note: trailer axle mid y-coordinate
  gp : Inport  PortDimensions=[1 3]
  semi_x : Inport  Port=2
  semi_y : Inport  Port=3
  i : Inport  Port=4  OutDataTypeStr=double
  theta_1 : Inport  Port=5
  gamma_1 : Inport  Port=6  OutDataTypeStr=double  PortDimensions=1
  Assignment1 : Assignment  NumberOfDimensions=3  DiagnosticForDimensions=Warning  IndexOptions=Index vector (port),Index vector (dialog),Index vector (port)  Indices=1,4,1  OutputSizes=1,1,1
  Assignment2 : Assignment  NumberOfDimensions=3  DiagnosticForDimensions=Warning  IndexOptions=Index vector (port),Index vector (dialog),Index vector (port)  Indices=1,1,1  OutputSizes=1,1,1
  Assignment3 : Assignment  NumberOfDimensions=3  DiagnosticForDimensions=Warning  IndexOptions=Index vector (port),Index vector (dialog),Index vector (port)  Indices=1,2,1  OutputSizes=1,1,1
  Assignment4 : Assignment  NumberOfDimensions=3  DiagnosticForDimensions=Warning  IndexOptions=Index vector (port),Index vector (dialog),Index vector (port)  Indices=1,3,1  OutputSizes=1,1,1
  Assignment5 : Assignment  NumberOfDimensions=2  DiagnosticForDimensions=Warning  IndexOptions=Index vector (port),Index vector (dialog)  Indices=1,1  OutputSizes=1,1
  Assignment6 : Assignment  NumberOfDimensions=2  DiagnosticForDimensions=Warning  IndexOptions=Index vector (port),Index vector (dialog)  Indices=1,1  OutputSizes=1,1
  Assignment7 : Assignment  NumberOfDimensions=2  DiagnosticForDimensions=Warning  IndexOptions=Index vector (port),Index vector (dialog)  Indices=1,2  OutputSizes=1,1
  Constant : Constant  Value=0
  Constant3 : Constant  Value=tstep
  Constant6 : Constant  Value=0
  Constant7 : Constant
  Data Store Read : DataStoreRead  DataStoreName=ip
  Data Store Read1 : DataStoreRead  DataStoreName=H  DataStoreElements=H.trajobtained(:,:,:)
  Data Store Read2 : DataStoreRead  DataStoreName=H  DataStoreElements=H.feasibility(:,:)
  Data Store Read3 : DataStoreRead  DataStoreName=H  DataStoreElements=H.inputgoalp(:,:)
  Data Store Write : DataStoreWrite  DataStoreName=H  DataStoreElements=H.trajobtained(:,:,:)
  Data Store Write1 : DataStoreWrite  DataStoreName=H  DataStoreElements=H.feasibility(:,:)
  Data Store Write2 : DataStoreWrite  DataStoreName=H  DataStoreElements=H.inputgoalp(:,:)
  Data Type Conversion : DataTypeConversion
  Delay1 : Delay  DelayLength=1
  Demux : Demux  Outputs=3
  Fcn : Fcn  Commented=on  Expr=sqrt(u(1)^2+u(2)^2)<=20
  Fcn1 : Fcn  Expr=sqrt((u(4)-u(1))^2+(u(5)-u(2))^2)
  Mux4 : Mux  Inputs=2
  OR : Logic  Operator=OR  IconShape=distinctive  AllPortsSameDT=off  OutDataTypeStr=boolean
  OR1 : Logic  Operator=OR  Inputs=3  IconShape=distinctive  AllPortsSameDT=off  OutDataTypeStr=boolean
  Relational Operator1 : RelationalOperator  Operator=<=  OutDataTypeStr=boolean  RndMeth=Simplest
  Resettable Subsystem : Subsystem  TreatAsAtomicUnit=on
  Switch : Switch  Criteria=u2 > Threshold
  Switch1 : Switch  Criteria=u2 > Threshold
  Switch3 : Switch  Threshold=indsimtime
  Terminator : Terminator
  checksfor_nan : MATLAB Function  TreatAsAtomicUnit=on
  excludeinfeasible_points : MATLAB Function  TreatAsAtomicUnit=on
  Out1 : Outport
  wires:
  Mux4/1 -> Fcn1/1
  Assignment3/1 -> Data Store Write/1
  Resettable Subsystem/1(Outport) -> Switch3/2, Assignment1/3, Assignment4/3, Assignment3/3, Assignment2/3
  Constant3/1 -> Relational Operator1/2
  Delay1/1 -> Resettable Subsystem/Reset
  Assignment1/1 -> Assignment2/1
  Assignment2/1 -> Assignment3/1
  Constant6/1 -> Switch3/3
  Constant7/1 -> Switch3/1
  Switch3/1 -> OR/2
  gp/1 -> Demux/1, excludeinfeasible_points/1(u), Mux4/1
  semi_y/1 -> Assignment3/2
  Relational Operator1/1 -> Delay1/1, OR/1
  Fcn1/1 -> Relational Operator1/1
  i/1 -> Assignment2/4, Assignment5/3, Assignment3/4, Assignment1/4, Assignment4/4, Assignment7/3, Assignment6/3
  Data Type Conversion/1 -> Out1/1
  semi_x/1 -> Assignment2/2
  Data Store Read1/1 -> Assignment4/1
  Assignment4/1 -> Assignment1/1
  theta_1/1 -> Assignment4/2
  Assignment6/1 -> Assignment7/1
  gamma_1/1 -> Assignment1/2
  Data Store Read2/1 -> Assignment5/1
  Assignment5/1 -> Data Store Write1/1
  Data Store Read3/1 -> Assignment6/1
  Demux/1 -> Assignment6/2
  Demux/2 -> Assignment7/2
  Assignment7/1 -> Data Store Write2/1
  Demux/3 -> Terminator/1
  OR1/1 -> Switch/2, Switch/1, Switch1/1, Switch1/2
  OR/1 -> Switch/3
  Switch/1 -> Data Type Conversion/1
  Constant/1 -> Switch1/3
  Switch1/1 -> Assignment5/2
  Data Store Read/1 -> checksfor_nan/1(u), Mux4/2
  checksfor_nan/1(y) -> OR1/3
  excludeinfeasible_points/1(y) -> OR1/1

== system hmapsf/Heuristic map for clrrt/propagateorForwardsimulationstage.propagate/Resettable Subsystem/KM/organizing Hmap_related data /Resettable Subsystem ==
  Reset : ResetPort  DisableCoverage=on
  Add1 : Sum
  Constant2 : Constant
  Counter Limited : simulink/Sources/Counter Limited  uplimit=indsimtime-1  tsamp=-1
  Outport : Outport
  wires:
  Counter Limited/1 -> Add1/1
  Constant2/1 -> Add1/2
  Add1/1 -> Outport/1

== stateflow chart hmapsf/Heuristic map for clrrt ==
  note: Implementation of the Heuristic map generating algorithm in STATEFLOW
  note: START
  state propagateorForwardsimulationstage
    en:
    %updateInitialConfigurationofcontrollerwithNn_ updating the
    %current vehicle position to controller. a linear reference line
    %is formed between the origin (0,0) at tn(Nn_) and gp_ a point
    %from the grgrid
    updateICofcont(Nn_);
    du:
    propagate(v_0,gp_,Nn_,k)
    %trans1 is the variable that indicates end of
    %individual forward simulation
    state propagate(v_0,gp,Nn_,i) [function]
    state updateICofcont(Nn_) [function]
  state savehmap
    %function that collects data like
    %individual grid point co-ordinates
    %and respective cost to build
    %heuristicmap
    ws();
    state ws [function]
  state extensioncostcalculation
    en:
    cost_cal(v_0,k);
  state stop [function]
  note: STOP
  note: k is used to index into the gridpoints array that has collection of all co-ordinates with -50m<=x<=50m & -50m<=y<=50m
      | with resolution of 0.5m; szp is the total number of gridpoints; propagate() forward simulates the vehiclemodel and
      | controller combination along the linear reference line formed between (0,0) at tn(Nn_,1:2),where tn is an array that stores
      | the co-ordinates from gridpoints and the respective extension cost, Nn_ is assigned value 1 where,tn(1,1:2)=(0,0);
      | trans1 is the variable that indicates end of individual forward simulation
  (junction 248) -> (junction 247) [order 1] : [k<=szp]
  (junction 247) -> propagateorForwardsimulationstage [order 2] : {gp_(1,1:2)=gridpoints(k,:);gp_(1,3)=0;}
  (junction 247) -> (junction 249) [order 1] : [k==11]
  (default) -> (junction 248) : {k=1;szp=size(gridpoints,1);}
  (junction 250) -> (junction 248)
  (junction 248) -> savehmap [order 2]
  propagateorForwardsimulationstage -> extensioncostcalculation : [trans1==1]
  savehmap -> (junction 251) : {stop;}
  (junction 249) -> (junction 250) : {k=k+1;}
  extensioncostcalculation -> (junction 249)
  data: v_0 function_input double size=1; gp function_input double size=[1 3]; Nn_ function_input double size=1; i function_input double size=1; Nn_ function_input double size=1; v_0_ function_input; i_ function_input; gp_ local double size=[1 3]; Nn_ local double size=[1 1] =1; k local; v_0 data_store_memory; trans1 data_store_memory; gridpoints data_store_memory; szp local; H data_store_memory
  function cost_cal(v_0_,i_):
    | function cost_cal(v_0_,i_)
    | global H
    | traj=H.trajobtained(:,1:4,i_);
    | ind_traj=find(traj(:,1));
    | sztraj=length(ind_traj);
    | cost = 0;
    | temp = 0;
    | if v_0_>0
    | for m = 2:sztraj+1
    |     temp = (10*(traj(m,1)-traj(m-1,1))^2+10*(traj(m,2)-traj(m-1,2))^2);   %based on "Motion Planning and Stabilization for a Reversing Truck and Trailer System" Oskar Ljungqvist
    |     cost = cost + temp;
    |   
    | end
    | 
    | elseif v_0_< 0
    | for m = 2:sztraj+1
    |     temp = (10*(traj(m,1)-traj(m-1,1))^2+10*(traj(m,2)-traj(m-1,2))^2+(10^4)*(traj(m,3)-traj(m-1,3))^2+(10^4)*(traj(m,4)-traj(m-1,4))^2);   %based on "Motion Planning and Stabilization for a Reversing Truck and Trailer System" Oskar Ljungqvist
    |     cost = cost + temp;
    |   
    | end
    | end
    | H.cost(i_,1)=cost;
    | end

== matlab function hmapsf/Heuristic map for clrrt/propagateorForwardsimulationstage.propagate/Resettable Subsystem/Controller/purepursuit_contrroller/func to calculate points of intersections ==
  data: gp input; Nn_ input; tn input; R input; P output; pos input
function P = calc_ips(gp, Nn_, tn, R,pos)
%this func calculates points of intersection between ref line (formed
%with goal point, start point) and look ahead circle with center at semitrailer axel midpoint  
P=zeros(2,2);
%
p1=gp;
p2=[tn(Nn_,1) tn(Nn_,2)];
slope = (p1(1,2)-p2(1,2))/(p1(1,1)-p2(1,1));
if slope == -inf || slope ==inf
    intercpt=p1(1,1);
else
intercpt = p2(1,2)-slope*p2(1,1);
end
%updating center of circle with the current pose of semitrailer axle
%position
centerx=pos(1,1);
centery=pos(2,1);
radius=R;
coder.extrinsic('linecirc')
[xout,yout] = linecirc(slope,intercpt,centerx,centery,radius);
P=[xout ; yout];

== matlab function hmapsf/Heuristic map for clrrt/propagateorForwardsimulationstage.propagate/Resettable Subsystem/Controller/purepursuit_contrroller/pure pursuit control law ==
  data: ip output; P input size=[2 2]; alpha output size=[1,1]; gp input size=[1 3]; L_1f input; yawangle_semi input; pos input; R input
function [ip,alpha] = controlleroutput(P,gp,L_1f,yawangle_semi,pos,R)
%this func calculates steer angle that pursues the ref line formed between
%start point and goal point chosen from wayp

Psz=size(P,2);          %num of intersection points, with x_cords in 1st column y_cords in 2nd column in matrix P
distarray=zeros(Psz,3); % intersection points distance to gp (goal point)
 for k=1:Psz
     distarray(k,1:2)=[P(1,k) P(2,k)];
     distarray(k,3)=sqrt((P(1,k)-gp(1,1))^2+(P(2,k)-gp(1,2))^2);
 end
%choosing the nearest intersection point to the goal point from the
%available 2 points of intersection between reference line and look ahead
%circle
sortP=sortrows(distarray,3);  
ip=sortP(1,1:2);
alpha=zeros(1,1);
%Theta_e
num=ip(1,1)-pos(1,1);
den=ip(1,2)-pos(2,1);
theta_e = atan2(den,num)-yawangle_semi;   %orientation error
alpha = -atan((2*L_1f*sin(theta_e))/R);   %steer angle that aims to reduce orientation error (please refer the thesis doc for graphical explaination)

== matlab function hmapsf/Heuristic map for clrrt/propagateorForwardsimulationstage.propagate/Resettable Subsystem/IK/IK_function ==
  data: x_1 input; y_1 input; theta_0 input; theta_1 input; x_1_dot output; gamma_virtual input; y_1_dot output; theta_0_dot output; theta_1_dot output; v_1 input; x_0f output; y_0f output; x_0 output; y_0 output; x_1f output; y_1f output; delta_C input; delta_I2K output; v_0 input
% The vehicle is described in global coordinates for which ISO system is used.
% Yaw rates can be derived from applying non-holonomic consraint (no lateral
% slip) on each axle.

function [x_1_dot,y_1_dot,theta_0_dot,theta_1_dot,x_0f,y_0f,x_0,y_0,x_1f,y_1f,...
         delta_I2K] = vehicle(x_1,y_1,theta_0,theta_1,gamma_virtual,v_1,delta_C, v_0)
     
L_0f = 3.8;  %(tractor wheelbase)
L_1f = 7.21; %(trailer wheel base)
L_0b = 0.48;
     %_______________________ position _________________________________________
%king-pin

        x_1f = x_1+L_1f*cos(theta_1);
        y_1f = y_1+L_1f*sin(theta_1);

 
% drive axle

        x_0 = x_1f-L_0b*cos(theta_0);
        y_0 = y_1f-L_0b*sin(theta_0);

% steer axle

        x_0f = x_0+L_0f*cos(theta_0);
        y_0f = y_0+L_0f*sin(theta_0);
                       
% yaw rate        
                                      
        theta_1_dot = abs(v_1)*tan(delta_C)/L_1f;                           % semitrailer
        theta_0_dot = sign(v_1)*sign(L_0b)*(-(v_1/L_0b)*sin(gamma_virtual)+...
                    (L_1f/L_0b)*(theta_1_dot)*cos(gamma_virtual));                % tractor 
                     
% semitrailer longitudinal velocity in its own local body coordinate system

       
        
        delta_I2K = atan(L_0f*theta_0_dot/v_0);
                    
        
%_________________________next iteration___________________________________
        
        x_1_dot = v_1 * cos(theta_1);                                       % tractor drive axle velocity in global x-direction
        y_1_dot = v_1 * sin(theta_1);                                       % tractor drive axle velocity in global y-direction

== matlab function hmapsf/Heuristic map for clrrt/propagateorForwardsimulationstage.propagate/Resettable Subsystem/KM/KM function ==
  data: x_0 input; y_0 input; theta_0 input; theta_1 input; x_0_dot output; L_0b parameter; L_1f parameter; y_0_dot output; theta_0_dot output; theta_1_dot output; v_0 input; x_0f output; y_0f output; x_1f output; y_1f output; x_1 output; y_1 output; gamma_1 output; v_1 output; delta input; L_0f parameter
% The vehicle is described in global coordinates for which ISO system is used.
% Yaw rates can be derived from applying non-holonomic consraint (no lateral
% slip) on each axle.

function [x_0_dot,y_0_dot,theta_0_dot,theta_1_dot,x_0f,y_0f,x_1f,y_1f,x_1,y_1,gamma_1,...
         v_1] = vehicle(x_0,y_0,theta_0,theta_1,L_0b, L_1f, v_0,delta, L_0f)
     
%_______________________ position _________________________________________
% steer axle

        x_0f = x_0+L_0f*cos(theta_0);
        y_0f = y_0+L_0f*sin(theta_0);
        
%king-pin

        x_1f = x_0+L_0b*cos(theta_0);
        y_1f = y_0+L_0b*sin(theta_0);
 
% semitrailer axle

        x_1 = x_1f-L_1f*cos(theta_1);
        y_1 = y_1f-L_1f*sin(theta_1);
        
% articulation angle
        
        gamma_1 = (theta_0-theta_1);                                        % articulation angle
        
% yaw rate        
        
        theta_0_dot = (v_0/L_0f) * tan(delta);                              % tractor 
        theta_1_dot = (v_0/L_1f)*sin(gamma_1) + (L_0b/L_1f)*...
                        (theta_0_dot)*cos(gamma_1);                         % semitrailer                            
                    
                    
% semitrailer longitudinal velocity in its own local body coordinate system

        v_1 = 1;  
                    
        
%_________________________next iteration____________________________________
        
        x_0_dot = v_0 * cos(theta_0);                                          % tractor drive axle velocity in global x-direction
        y_0_dot = v_0 * sin(theta_0);                                          % tractor drive axle velocity in global y-direction

== matlab function hmapsf/Heuristic map for clrrt/propagateorForwardsimulationstage.propagate/Resettable Subsystem/KM/organizing Hmap_related data /checksfor_nan ==
  data: u input; y output
function y = fcn(u)
if any(isnan(u), 'all')
    y=1;
else
    y=0;
end

== matlab function hmapsf/Heuristic map for clrrt/propagateorForwardsimulationstage.propagate/Resettable Subsystem/KM/organizing Hmap_related data /excludeinfeasible_points ==
  data: u input; y output; v_0 data_store_memory
function y = fcn(u)
global v_0
y=0;
if v_0>0
    if u(1,1)==0 && any(u(1,2)==-50:5:0)
        y=1;
    else
        y=0;
    end
elseif v_0<0
    if u(1,1)==0 && any(u(1,2)==0:5:50)
        y=1;
    else
        y=0;
    end
end

== matlab function hmapsf/Heuristic map for clrrt/propagateorForwardsimulationstage.updateICofcont/MATLAB Function ==
  data: IC_x1 output; IC_y1 output; Nn_ input; IC_x0 output; tn input; IC_y0 output; IC_theta0 output; IC_theta1 output
function [IC_x1,IC_y1,IC_x0,IC_y0,IC_theta0,IC_theta1] = fcn(Nn_,tn)
Nn=[tn(Nn_,1) tn(Nn_,2) tn(Nn_,9) tn(Nn_,10)];
L_0f = 3.8;  %(tractor wheelbase)
L_1f = 7.21; %(trailer wheel base)
L_0b = 0.48;
        %updating the vehicle position to controller
                IC_x1= 0+Nn(1,1);                                                         % initial x-position of semi axle 
                IC_y1 = 0+Nn(1,2);
                IC_theta0 = Nn(1,3);                                                   % initial yaw angle of tractor [deg]
                IC_theta1 = Nn(1,4);
                
                IC_x1f= L_1f*cos(IC_theta1)+IC_x1 ;                                                         % initial x-position of semi axle 
                IC_y1f =L_1f*sin(IC_theta1)+IC_y1 ;
                
                IC_x0f= (L_0f-L_0b)*cos(IC_theta0)+IC_x1f ;                                                         % initial x-position of semi axle 
                IC_y0f =(L_0f-L_0b)*sin(IC_theta0)+IC_y1f ;
                
                IC_x0 =   IC_x0f-L_0f*cos(IC_theta0);                                                           % initial x-position of tractor drive axle 
                IC_y0 =   IC_y0f-L_0f*sin(IC_theta0);
